simulink model "TwoTanksSystem_slx_org"  (Simulink 10.0)
settings: Solver=ode45  StartTime=0.0  StopTime=10  RelTol=1e-3  EnableMultiTasking=on
settings Model: Creator=zhangpn  LastModifiedBy=annonymous
settings DataIOCC: LimitDataPoints=on
settings DebuggingCC: SolverPrmCheckMsg=warning  StateNameClashWarn=warning
settings GRTTargetCC: GeneratePreprocessorConditionals=Disable all  CombineOutputUpdateFcns=on  GRTInterface=off
settings ConfigComp: CovExternalEMLEnable=off

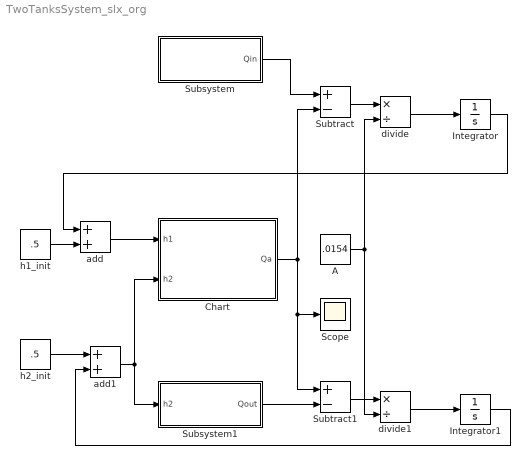
== system TwoTanksSystem_slx_org ==
  A : Constant  Value=.0154
  Chart : Stateflow chart  TreatAsAtomicUnit=on
  Integrator : Integrator
  Integrator1 : Integrator
  Scope : Scope
  Subsystem : Subsystem
  Subsystem1 : Subsystem
  Subtract : Sum  Inputs=+-
  Subtract1 : Sum  Inputs=+-
  add : Sum
  add1 : Sum
  divide : Product  Inputs=*/
  divide1 : Product  Inputs=*/
  h1_init : Constant  Value=.5
  h2_init : Constant  Value=.5
  wires:
  Subsystem/1(Qin) -> Subtract/1
  Subsystem1/1(Qout) -> Subtract1/2
  Chart/1(Qa) -> Scope/1, Subtract1/1, Subtract/2
  Subtract/1 -> divide/1
  A/1 -> divide/2, divide1/2
  Subtract1/1 -> divide1/1
  divide/1 -> Integrator/1
  divide1/1 -> Integrator1/1
  Integrator/1 -> add/1
  h1_init/1 -> add/2
  add/1 -> Chart/1(h1)
  h2_init/1 -> add1/1
  Integrator1/1 -> add1/2
  add1/1 -> Subsystem1/1(h2), Chart/2(h2)

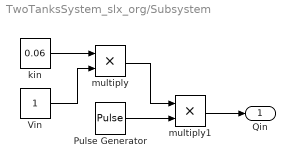
== system TwoTanksSystem_slx_org/Subsystem ==
  Pulse Generator : DiscretePulseGenerator  PulseType=Time based  Period=1  PulseWidth=50
  Vin : Constant
  kin : Constant  Value=0.06
  multiply : Product  Inputs=**
  multiply1 : Product  Inputs=**
  Qin : Outport
  wires:
  Vin/1 -> multiply/2
  multiply/1 -> multiply1/1
  Pulse Generator/1 -> multiply1/2
  kin/1 -> multiply/1
  multiply1/1 -> Qin/1

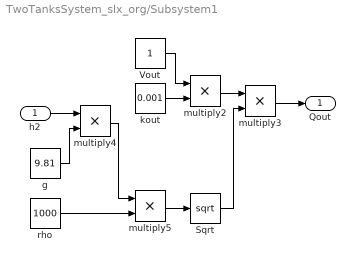
== system TwoTanksSystem_slx_org/Subsystem1 ==
  h2 : Inport
  Sqrt : Sqrt  SaturateOnIntegerOverflow=on
  Vout : Constant
  g : Constant  Value=9.81
  kout : Constant  Value=0.001
  multiply{2..5} (4 alike) : Product  Inputs=**
  rho : Constant  Value=1000
  Qout : Outport
  wires:
  multiply3/1 -> Qout/1
  kout/1 -> multiply2/2
  multiply2/1 -> multiply3/1
  h2/1 -> multiply4/1
  g/1 -> multiply4/2
  multiply4/1 -> multiply5/1
  rho/1 -> multiply5/2
  multiply5/1 -> Sqrt/1
  Sqrt/1 -> multiply3/2
  Vout/1 -> multiply2/1

== stateflow chart Chart ==
  state level1
    entry: Qa = 0;
  state level3
    entry: Qa = -Va * Ka * sqrt(p*g*(h2-h));
  state Init
  state level2
    entry: Qa = Va * Ka * sqrt(p*g*(h1-h));
  state level4
    entry: Qa = Sign(h1, h2)*Va*Ka*sqrt(p*g*abs(h1-h2));
  level3 -> level1 [order 1] : [h1 < h & h2 < h]
  level4 -> level1 [order 3] : [h1 < h & h2 < h]
  level1 -> level3 [order 1] : [h1 < h & h2 > h]
  Init -> level1 [order 1] : [h1 < h & h2 < h]
  Init -> level3 [order 2] : [h1 < h & h2 > h]
  level2 -> level1 [order 1] : [h1 < h & h2 < h]
  level1 -> level2 [order 2] : [h1 >= h & h2 <= h]
  level1 -> level4 [order 3] : [h1 > h & h2 > h]
  level2 -> level3 [order 2] : [h1 < h & h2 > h]
  level3 -> level2 [order 2] : [h1 >= h & h2 <= h]
  level4 -> level3 [order 2] : [h1 < h & h2 > h]
  level3 -> level4 [order 3] : [h1 > h & h2 > h]
  (default) -> Init
  Init -> level2 [order 3] : [h1 >= h & h2 <= h]
  Init -> level4 [order 4] : [h1 > h & h2 > h]
  level2 -> level4 [order 3] : [h1 > h & h2 > h]
  level4 -> level2 [order 1] : [h1 >= h & h2 <= h]
  data: x1 function_input double; x2 function_input double; sign function_output double; Qa output double; Va constant double =1; Ka constant double =0.001; rho constant double =1000; g constant double =9.81; h constant double =0.3; h1 input double; h2 input double
  function sign = Sign(x1,x2):
    | function sign = Sign(x1,x2)
    | if (x1 > x2)
    |     sign = 1;
    | elseif (x1 < x2)
    |     sign = -1; 
    | else
    |     sign = 0;
    | end
